simulink model "mdllogisti"  (Simulink 7.8)
settings: Solver=ode45  StartTime=0.0  StopTime=100  RelTol=1e-3
settings Model: Creator=polacmi1  LastModifiedBy=polacekm
settings GRTTargetCC: CombineOutputUpdateFcns=on

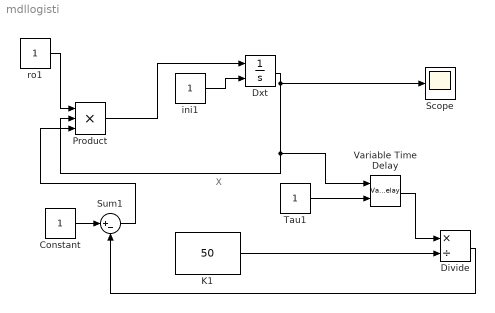
== system mdllogisti ==
  note: X
  Constant : Constant
  Divide : Product  Inputs=*/
  Dxt : Integrator  InitialConditionSource=external  InitialCondition=1
  K1 : Constant  Value=50
  Product : Product  Inputs=3  RndMeth=Zero
  Scope : Scope
      settings: SaveName=sc
  Sum1 : Sum  Inputs=|+-
  Tau1 : Constant
  Variable Time Delay : VariableTransportDelay  MaximumDelay=10
  ini1 : Constant
  ro1 : Constant
  wires:
  Dxt/1 -> Product/2, Variable Time Delay/1, Scope/1
  ro1/1 -> Product/1
  Product/1 -> Dxt/1
  Constant/1 -> Sum1/1
  K1/1 -> Divide/2
  Divide/1 -> Sum1/2
  Sum1/1 -> Product/3
  Tau1/1 -> Variable Time Delay/2
  Variable Time Delay/1 -> Divide/1
  ini1/1 -> Dxt/2
